simulink model "gm_sampleModel2003_2_sub_sub_sub"  (R2023a)
settings: Solver=VariableStepAuto  StartTime=0.0  StopTime=10.0  RelTol=1e-3
libraries: hdlsllib x7, simulink x2
settings Model: Creator=user1  LastModifiedBy=user1
settings OptimizationCC: BlockReduction=off  ConditionallyExecuteInputs=off
settings DebuggingCC: InheritedTsInSrcMsg=none

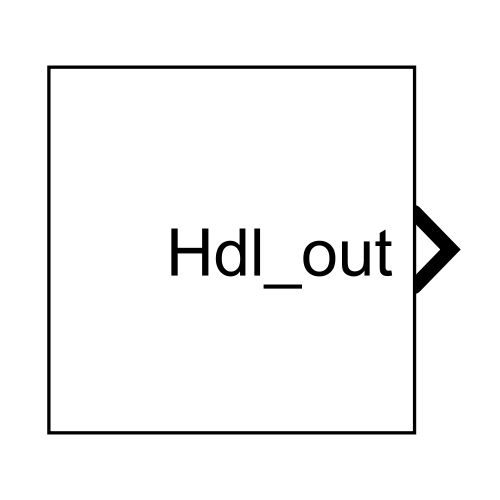
[thumbnail: Simulink's stored preview of the top-level diagram]
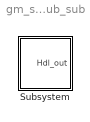
== system gm_sampleModel2003_2_sub_sub_sub ==
  Subsystem : Subsystem

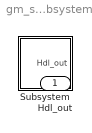
== system gm_sampleModel2003_2_sub_sub_sub/Subsystem ==
  Subsystem : Subsystem
  Hdl_out : Outport  OutDataTypeStr=uint8

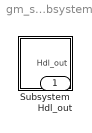
== system gm_sampleModel2003_2_sub_sub_sub/Subsystem/Subsystem ==
  Subsystem : Subsystem
  Hdl_out : Outport  OutDataTypeStr=uint8

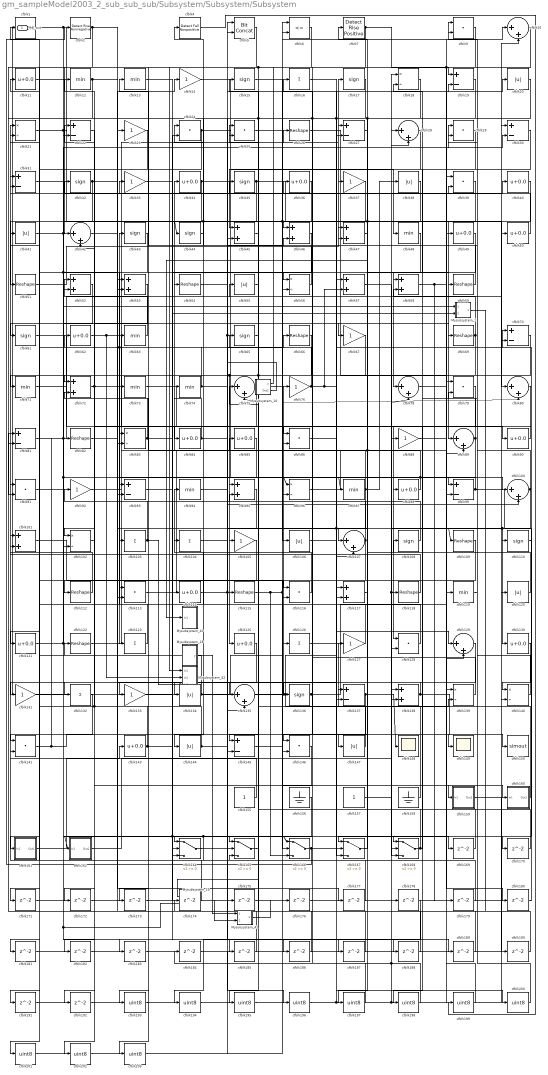
== system gm_sampleModel2003_2_sub_sub_sub/Subsystem/Subsystem/Subsystem ==
  Mysubsystem_1 : Subsystem  TreatAsAtomicUnit=on  RTWFcnName=Mysubsystem_1
      settings: RTWFcnNameOpts=User specified  RTWFileNameOpts=Use function name
  Mysubsystem_10 : Subsystem  TreatAsAtomicUnit=on  RTWFcnName=Mysubsystem_10
      settings: RTWFcnNameOpts=User specified  RTWFileNameOpts=Use function name
  Mysubsystem_28 : Subsystem  TreatAsAtomicUnit=on  RTWFcnName=Mysubsystem_28
      settings: RTWFcnNameOpts=User specified  RTWFileNameOpts=Use function name
  Mysubsystem_29 : Subsystem  TreatAsAtomicUnit=on  RTWFcnName=Mysubsystem_29
      settings: RTWFcnNameOpts=User specified  RTWFileNameOpts=Use function name
  Mysubsystem_40 : Subsystem  TreatAsAtomicUnit=on  RTWFcnName=Mysubsystem_40
      settings: RTWFcnNameOpts=User specified  RTWFileNameOpts=Use function name
  Mysubsystem_41 : Subsystem  TreatAsAtomicUnit=on  RTWFcnName=Mysubsystem_41
      settings: RTWFcnNameOpts=User specified  RTWFileNameOpts=Use function name
  Mysubsystem_42 : Subsystem  TreatAsAtomicUnit=on  RTWFcnName=Mysubsystem_42
      settings: RTWFcnNameOpts=User specified  RTWFileNameOpts=Use function name
  cfblk1 : hdlsllib/Logic and Bit Operations/Compare To Constant  relop=<=  const=3.0  OutDataTypeStr=uint8
  cfblk{10,28,42,75,78,80,89,100,107,129,135} (11 alike) : Sum  Inputs=|++  OutDataTypeStr=uint8
  cfblk{45..47,52..53,57..58,72,95,101,117,138} (12 alike) : Sum  OutDataTypeStr=uint8
  cfblk{18,21,56,83,96,102,139..140} (8 alike) : Product  Inputs=*/  OutDataTypeStr=uint8  RndMeth=Zero  SaturateOnIntegerOverflow=on
  cfblk{16,103..104,123,126,132} (6 alike) : Sum  Inputs=+  OutDataTypeStr=uint8
  cfblk{14,23,33,37,67,76,88,92,105,127,131,133} (12 alike) : Gain  OutDataTypeStr=uint8
  cfblk{20,38,41,55,106,120,134,144,147} (9 alike) : Abs  OutDataTypeStr=uint8  SaturateOnIntegerOverflow=off
  cfblk{15,17,32,35,43..44,61,65,108,110,136} (11 alike) : Signum
  cfblk{26,51,54,59,66,69,82,109,112,115,118,122} (12 alike) : Reshape
  cfblk{11,34,36,40,49..50,62,84..85,90,98,114,121,125,130,143} (16 alike) : Bias  Bias=0.0  SaturateOnIntegerOverflow=off
  cfblk{9,24..25,29,39,79,86,91,113,116,128,141,146} (13 alike) : DotProduct  OutDataTypeStr=uint8
  cfblk{12..13,48,63,71,73..74,94,97,119} (10 alike) : MinMax  OutDataTypeStr=uint8
  cfblk{19,22,27,30..31,70,81,93,99,137,145} (11 alike) : Sum  Inputs=+-  OutDataTypeStr=uint8
  cfblk148 : Scope
  cfblk149 : Scope
  cfblk150 : ToWorkspace  VariableName=simout  SaveFormat=Timeseries  SampleTime=-1
  cfblk155 : Constant  OutDataTypeStr=uint8  SampleTime=-1
  cfblk156 : Ground
  cfblk157 : Constant  OutDataTypeStr=uint8  SampleTime=-1
  cfblk158 : Ground
  cfblk159 : Subsystem
      settings: LibrarySourceBlock=|
      | hdlsllib/Ports &
      | Subsystems/Subsystem
  cfblk160 : Subsystem
      settings: LibrarySourceBlock=|
      | hdlsllib/Ports &
      | Subsystems/Subsystem
  cfblk161 : Subsystem
      settings: LibrarySourceBlock=|
      | hdlsllib/Ports &
      | Subsystems/Subsystem
  cfblk162 : Subsystem
      settings: LibrarySourceBlock=|
      | hdlsllib/Ports &
      | Subsystems/Subsystem
  cfblk{164..168} (5 alike) : Switch  OutDataTypeStr=uint8  SaturateOnIntegerOverflow=off  InputSameDT=off
  cfblk{169..192} (24 alike) : Delay  SampleTime=1
  cfblk{193..203} (11 alike) : DataTypeConversion  OutDataTypeStr=uint8  SaturateOnIntegerOverflow=off  RndMeth=Floor
  cfblk2 : hdlsllib/Logic and Bit Operations/Detect Rise Nonnegative  vinit=0  OutDataTypeStr=uint8
  cfblk4 : hdlsllib/Logic and Bit Operations/Detect Fall Nonpositive  vinit=0  OutDataTypeStr=uint8
  cfblk5 : hdlsllib/Logic and Bit Operations/Bit Concat  numInputs=2
  cfblk6 : RelationalOperator  Operator=<=  OutDataTypeStr=boolean  InputSameDT=off
  cfblk7 : hdlsllib/Logic and Bit Operations/Detect Rise Positive  vinit=0  OutDataTypeStr=uint8
  Hdl_out : Outport  OutDataTypeStr=uint8
  wires:
  Mysubsystem_41/1(Out1) -> cfblk178/1
  Mysubsystem_29/1(Out1) -> Mysubsystem_41/2(In2)
  Mysubsystem_28/1(y) -> Mysubsystem_41/1(In1)
  Mysubsystem_10/2(Out2) -> cfblk100/1, cfblk20/1
  Mysubsystem_10/1(y) -> Mysubsystem_42/1(In1), cfblk145/1
  Mysubsystem_1/1(Out1) -> cfblk174/1
  cfblk203/1 -> cfblk5/2
  cfblk202/1 -> cfblk5/1
  cfblk146/1 -> cfblk202/1
  cfblk201/1 -> cfblk176/1
  cfblk5/1 -> cfblk201/1
  cfblk200/1 -> cfblk79/2
  cfblk196/1 -> cfblk200/1
  cfblk199/1 -> cfblk79/1
  cfblk4/1 -> cfblk199/1
  cfblk198/1 -> cfblk86/2, cfblk18/1
  cfblk197/1 -> cfblk184/1
  cfblk49/1 -> cfblk197/1
  cfblk184/1 -> cfblk196/1
  cfblk195/1 -> cfblk6/2
  cfblk165/1 -> cfblk195/1
  cfblk194/1 -> cfblk6/1
  cfblk178/1 -> cfblk194/1
  cfblk193/1 -> cfblk118/1, cfblk78/2, cfblk120/1, cfblk57/1
  cfblk192/1 -> cfblk165/2
  cfblk191/1 -> cfblk139/1
  cfblk109/1 -> cfblk191/1
  cfblk190/1 -> cfblk116/2
  cfblk159/1(Out1) -> cfblk190/1
  cfblk189/1 -> cfblk168/2
  cfblk131/1 -> cfblk189/1
  cfblk188/1 -> cfblk167/2
  cfblk187/1 -> cfblk81/1
  cfblk27/1 -> cfblk187/1
  cfblk186/1 -> cfblk165/3
  cfblk185/1 -> cfblk53/1
  cfblk91/1 -> cfblk185/1
  cfblk183/1 -> cfblk140/2
  cfblk182/1 -> cfblk30/1
  cfblk105/1 -> cfblk182/1
  cfblk181/1 -> cfblk117/1
  cfblk23/1 -> cfblk181/1
  cfblk180/1 -> cfblk70/2
  cfblk179/1 -> cfblk141/2
  cfblk177/1 -> cfblk75/1
  cfblk176/1 -> cfblk96/2
  cfblk175/1 -> cfblk39/1
  cfblk164/1 -> cfblk175/1
  cfblk174/1 -> cfblk1/1
  cfblk173/1 -> cfblk89/2
  cfblk129/1 -> cfblk173/1
  cfblk172/1 -> cfblk24/2
  cfblk171/1 -> cfblk10/2
  cfblk132/1 -> cfblk171/1
  cfblk170/1 -> cfblk95/2
  cfblk110/1 -> cfblk170/1
  cfblk169/1 -> cfblk18/2
  cfblk57/1 -> cfblk169/1
  cfblk101/1 -> cfblk166/2
  cfblk65/1 -> cfblk15/1
  cfblk58/1 -> cfblk179/1, cfblk180/1
  cfblk6/1 -> cfblk193/1
  cfblk29/1 -> cfblk58/1
  cfblk36/1 -> cfblk52/2
  cfblk74/1 -> cfblk62/1, cfblk135/2
  cfblk160/1(Out1) -> cfblk32/1
  cfblk158/1 -> cfblk137/1
  cfblk41/1 -> cfblk69/1, cfblk30/2
  cfblk83/1 -> cfblk166/1, cfblk186/1, cfblk72/2
  cfblk54/1 -> cfblk110/1
  cfblk138/1 -> cfblk150/1, cfblk136/1
  cfblk55/1 -> cfblk25/1
  cfblk67/1 -> cfblk72/1
  cfblk104/1 -> cfblk46/2
  cfblk22/1 -> cfblk102/1
  cfblk127/1 -> cfblk104/1
  cfblk14/1 -> cfblk48/1
  cfblk108/1 -> cfblk35/1
  cfblk15/1 -> cfblk90/1
  cfblk119/1 -> cfblk29/1
  cfblk28/1 -> cfblk45/1
  cfblk144/1 -> cfblk122/1, cfblk31/1, cfblk27/1
  cfblk73/1 -> cfblk129/2
  cfblk145/1 -> cfblk9/2
  cfblk114/1 -> cfblk29/2, cfblk188/1
  cfblk12/1 -> cfblk23/1, cfblk22/2
  cfblk10/1 -> cfblk75/2, cfblk91/2
  cfblk93/1 -> cfblk164/2
  cfblk13/1 -> cfblk67/1
  cfblk115/1 -> cfblk159/1(In1), cfblk80/2, cfblk166/3
  cfblk123/1 -> cfblk41/1
  cfblk45/1 -> cfblk165/1
  cfblk125/1 -> cfblk141/1
  cfblk9/1 -> cfblk61/1, cfblk99/2
  cfblk116/1 -> cfblk94/1
  cfblk47/1 -> cfblk147/1
  cfblk71/1 -> cfblk50/1
  cfblk168/1 -> cfblk65/1, cfblk108/1
  cfblk82/1 -> cfblk14/1
  cfblk69/1 -> Mysubsystem_29/1(In1), cfblk103/1, cfblk58/2
  cfblk84/1 -> cfblk66/1, cfblk74/1
  cfblk75/1 -> cfblk99/1, cfblk192/1
  cfblk20/1 -> cfblk146/1
  cfblk78/1 -> cfblk10/1
  cfblk21/1 -> cfblk183/1, Mysubsystem_29/2(In2), cfblk46/1
  cfblk167/1 -> cfblk37/1
  cfblk31/1 -> cfblk114/1
  cfblk147/1 -> cfblk127/1
  cfblk16/1 -> cfblk168/1, cfblk109/1
  cfblk37/1 -> cfblk51/1
  cfblk92/1 -> cfblk85/1
  cfblk76/1 -> cfblk19/2, cfblk57/2, cfblk63/1, cfblk31/2
  cfblk32/1 -> cfblk102/2, cfblk177/1
  cfblk140/1 -> cfblk9/1
  cfblk33/1 -> cfblk59/1
  cfblk118/1 -> cfblk101/2
  cfblk94/1 -> cfblk100/2
  cfblk141/1 -> cfblk149/1, cfblk82/1
  cfblk130/1 -> cfblk140/1
  cfblk139/1 -> cfblk16/1
  cfblk95/1 -> cfblk133/1
  cfblk89/1 -> cfblk33/1, cfblk167/3
  cfblk143/1 -> Mysubsystem_1/2(In2), cfblk42/2
  cfblk62/1 -> Mysubsystem_42/2(In2), cfblk115/1
  cfblk157/1 -> cfblk28/2
  cfblk11/1 -> cfblk97/1, cfblk164/3, cfblk53/2
  cfblk61/1 -> cfblk86/1
  cfblk90/1 -> cfblk83/1
  cfblk162/1(Out1) -> cfblk138/2
  cfblk81/1 -> cfblk55/1, cfblk36/1
  cfblk70/1 -> cfblk71/1
  cfblk155/1 -> cfblk101/1
  cfblk79/1 -> cfblk198/1
  cfblk7/1 -> cfblk56/1, cfblk19/1
  cfblk102/1 -> cfblk132/1
  cfblk39/1 -> cfblk44/1, cfblk56/2
  cfblk133/1 -> cfblk39/2
  cfblk98/1 -> cfblk73/1, cfblk47/1, cfblk96/1
  cfblk24/1 -> cfblk117/2, cfblk83/2
  cfblk72/1 -> cfblk54/1, cfblk22/1
  cfblk34/1 -> cfblk138/1, cfblk203/1
  cfblk100/1 -> cfblk130/1, cfblk128/2, cfblk47/2
  cfblk137/1 -> cfblk148/1, cfblk146/2
  cfblk136/1 -> cfblk88/1, Hdl_out/1
  cfblk96/1 -> cfblk28/1
  cfblk117/1 -> cfblk7/1
  cfblk113/1 -> cfblk40/1
  cfblk86/1 -> cfblk98/1
  cfblk50/1 -> cfblk11/1
  cfblk43/1 -> cfblk131/1
  cfblk63/1 -> cfblk52/1
  cfblk40/1 -> Mysubsystem_40/1(In1), cfblk161/1(In1)
  cfblk134/1 -> cfblk21/2, cfblk126/1
  cfblk48/1 -> cfblk78/1
  cfblk88/1 -> cfblk160/1(In1)
  cfblk80/1 -> cfblk128/1
  cfblk52/1 -> cfblk121/1
  cfblk166/1 -> cfblk2/1, cfblk70/1
  cfblk99/1 -> cfblk167/1, cfblk93/1
  cfblk53/1 -> cfblk112/1
  cfblk59/1 -> cfblk4/1
  cfblk56/1 -> cfblk13/1
  cfblk106/1 -> cfblk129/1
  cfblk46/1 -> cfblk123/1
  cfblk103/1 -> Mysubsystem_42/3(In3), cfblk12/1
  cfblk25/1 -> cfblk106/1
  cfblk18/1 -> cfblk116/1, cfblk145/2, cfblk27/2
  cfblk30/1 -> cfblk105/1
  cfblk42/1 -> cfblk164/1
  cfblk112/1 -> cfblk91/1
  cfblk66/1 -> cfblk95/1, cfblk93/2
  cfblk107/1 -> cfblk25/2, cfblk172/1
  cfblk120/1 -> cfblk92/1
  cfblk26/1 -> cfblk119/1
  cfblk85/1 -> cfblk125/1
  cfblk156/1 -> cfblk21/1, cfblk162/1(In1)
  cfblk135/1 -> cfblk139/2, cfblk107/2, cfblk76/1
  cfblk51/1 -> cfblk17/1
  cfblk38/1 -> cfblk134/1
  cfblk44/1 -> cfblk24/1
  cfblk161/1(Out1) -> cfblk143/1
  cfblk128/1 -> cfblk43/1
  cfblk19/1 -> cfblk107/1, cfblk81/2
  cfblk126/1 -> cfblk49/1
  cfblk35/1 -> cfblk144/1, cfblk113/1, cfblk80/1
  cfblk17/1 -> cfblk84/1, cfblk135/1
  cfblk1/1 -> cfblk89/1, cfblk45/2
  cfblk122/1 -> cfblk26/1
  cfblk121/1 -> Mysubsystem_1/1(In1), cfblk168/3
  cfblk97/1 -> cfblk34/1, cfblk38/1, cfblk113/2
  cfblk2/1 -> cfblk42/1, cfblk137/2

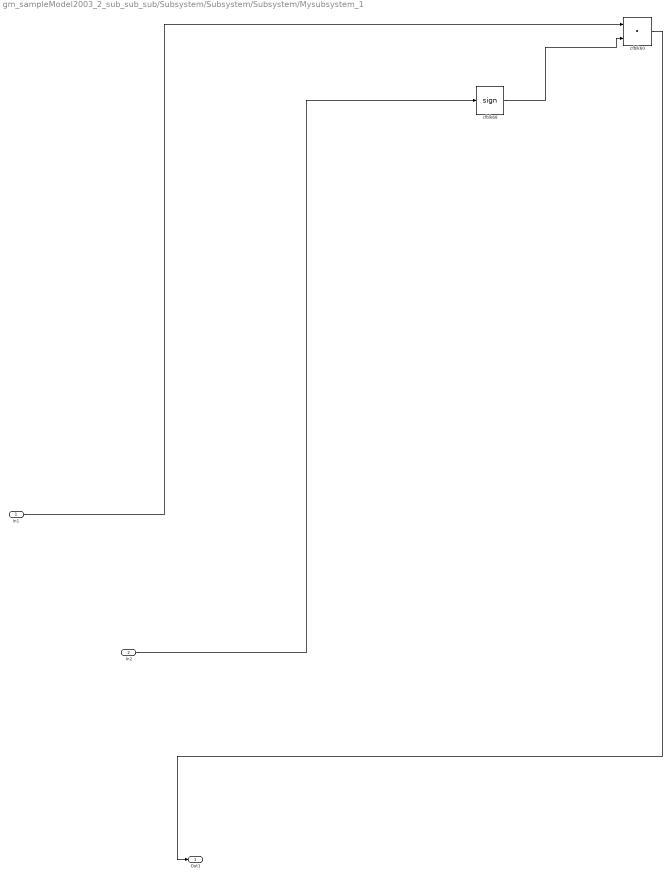
== system gm_sampleModel2003_2_sub_sub_sub/Subsystem/Subsystem/Subsystem/Mysubsystem_1 ==
  In1 : Inport
  In2 : Inport  Port=2
  cfblk60 : DotProduct  OutDataTypeStr=Inherit: Inherit via internal rule
  cfblk68 : Signum
  Out1 : Outport
  wires:
  cfblk68/1 -> cfblk60/2
  In1/1 -> cfblk60/1
  cfblk60/1 -> Out1/1
  In2/1 -> cfblk68/1

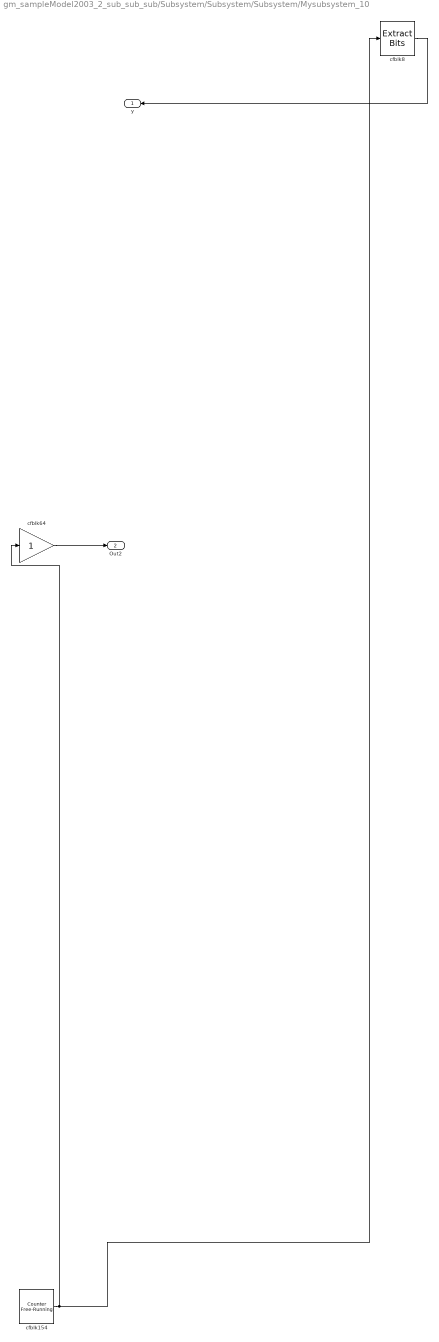
== system gm_sampleModel2003_2_sub_sub_sub/Subsystem/Subsystem/Subsystem/Mysubsystem_10 ==
  cfblk154 : hdlsllib/Sources/Counter Free-Running  NumBits=16  tsamp=-1
  cfblk64 : Gain
  cfblk8 : simulink/Logic and Bit Operations/Extract Bits  bitsToExtract=Upper half  numBits=8  bitIdxRange=[0 7]  outScalingMode=Preserve fixed-point scaling
      settings: LibrarySourceBlock=|
      | hdlsllib/Logic and Bit
      | Operations/Extract Bits
  y : Outport
  Out2 : Outport  Port=2
  wires:
  cfblk64/1 -> Out2/1
  cfblk8/1 -> y/1
  cfblk154/1 -> cfblk8/1, cfblk64/1

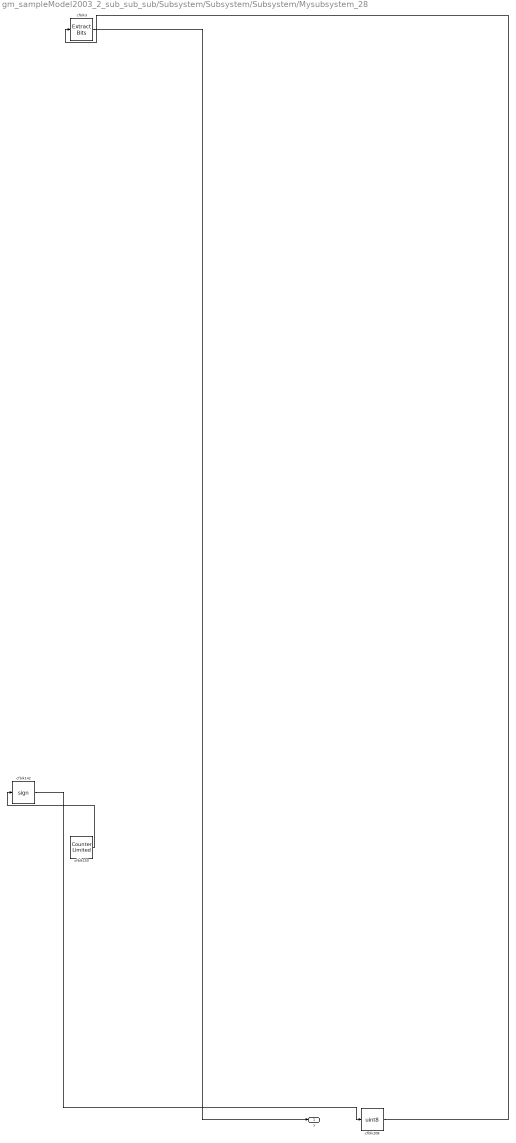
== system gm_sampleModel2003_2_sub_sub_sub/Subsystem/Subsystem/Subsystem/Mysubsystem_28 ==
  cfblk142 : Signum
  cfblk153 : hdlsllib/Sources/Counter Limited  uplimit=7  tsamp=-1
  cfblk208 : DataTypeConversion  OutDataTypeStr=uint8  SaturateOnIntegerOverflow=off  RndMeth=Floor
  cfblk3 : simulink/Logic and Bit Operations/Extract Bits  bitsToExtract=Upper half  numBits=8  bitIdxRange=[0 7]  outScalingMode=Preserve fixed-point scaling
      settings: LibrarySourceBlock=|
      | hdlsllib/Logic and Bit
      | Operations/Extract Bits
  y : Outport
  wires:
  cfblk142/1 -> cfblk208/1
  cfblk208/1 -> cfblk3/1
  cfblk3/1 -> y/1
  cfblk153/1 -> cfblk142/1

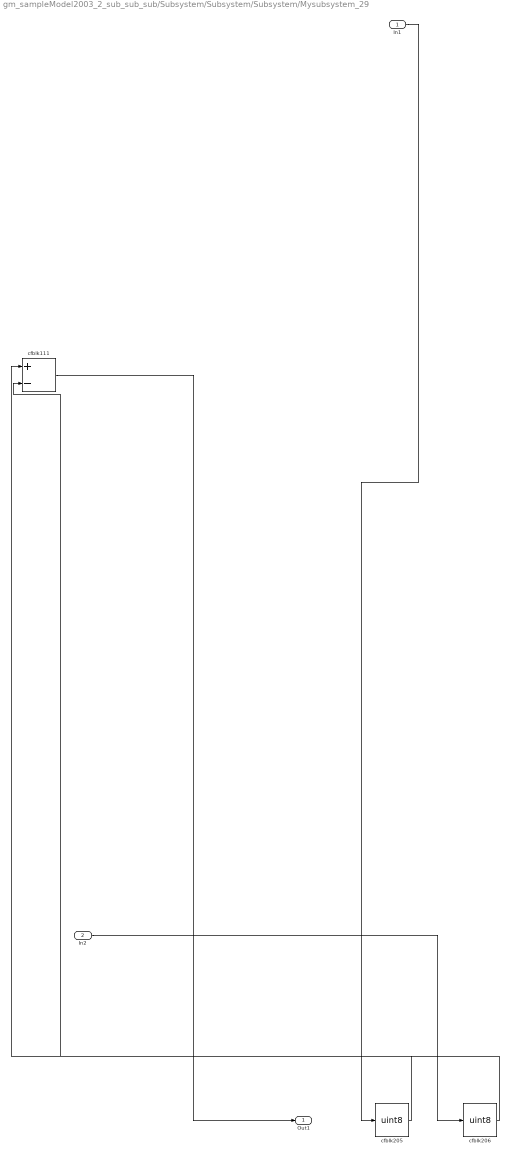
== system gm_sampleModel2003_2_sub_sub_sub/Subsystem/Subsystem/Subsystem/Mysubsystem_29 ==
  In1 : Inport
  In2 : Inport  Port=2
  cfblk111 : Sum  Inputs=+-
  cfblk205 : DataTypeConversion  OutDataTypeStr=uint8  SaturateOnIntegerOverflow=off  RndMeth=Floor
  cfblk206 : DataTypeConversion  OutDataTypeStr=uint8  SaturateOnIntegerOverflow=off  RndMeth=Floor
  Out1 : Outport
  wires:
  cfblk206/1 -> cfblk111/2
  In2/1 -> cfblk206/1
  In1/1 -> cfblk205/1
  cfblk205/1 -> cfblk111/1
  cfblk111/1 -> Out1/1

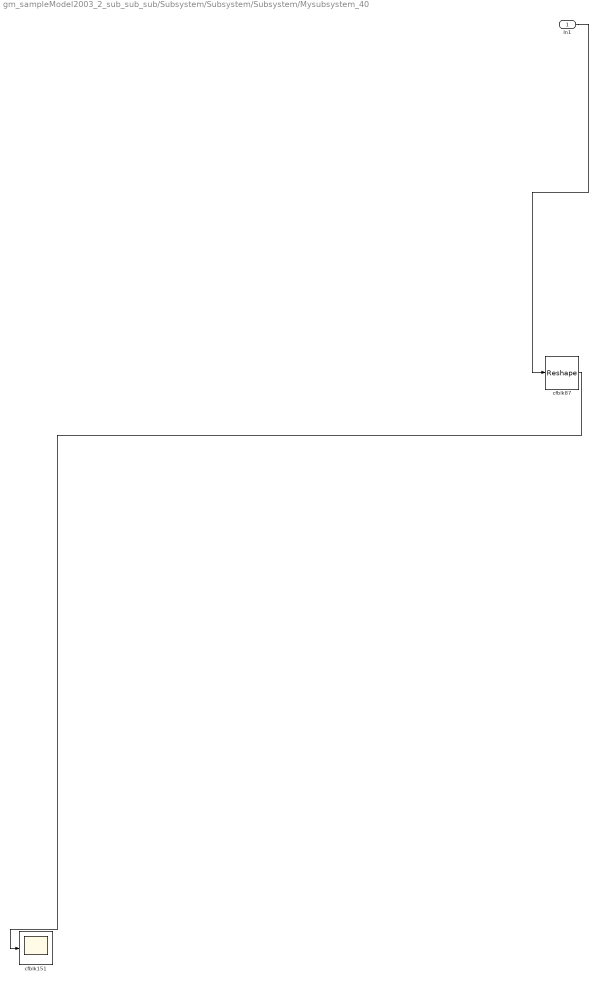
== system gm_sampleModel2003_2_sub_sub_sub/Subsystem/Subsystem/Subsystem/Mysubsystem_40 ==
  In1 : Inport
  cfblk151 : Scope
  cfblk87 : Reshape
  wires:
  In1/1 -> cfblk87/1
  cfblk87/1 -> cfblk151/1

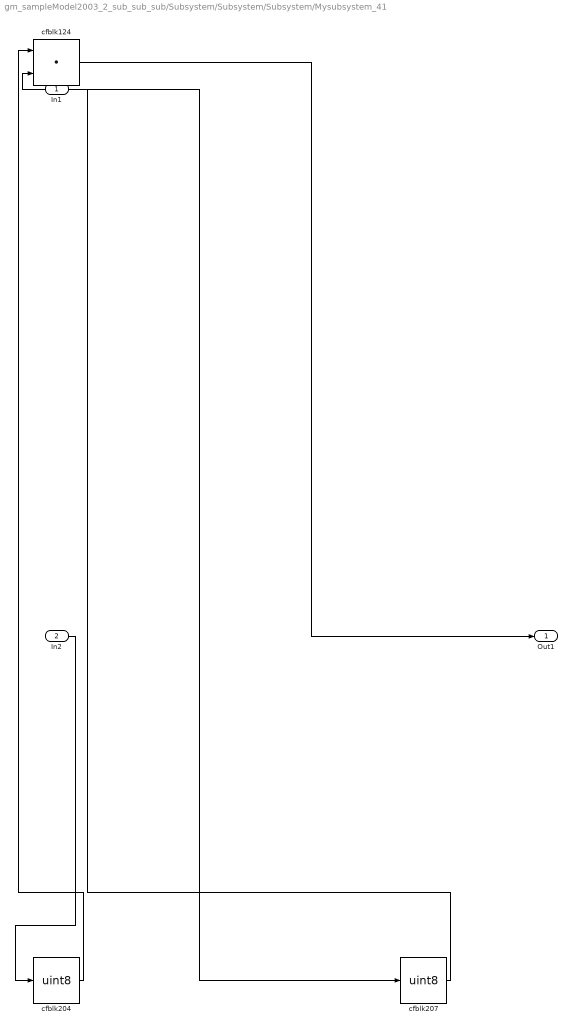
== system gm_sampleModel2003_2_sub_sub_sub/Subsystem/Subsystem/Subsystem/Mysubsystem_41 ==
  In1 : Inport
  In2 : Inport  Port=2
  cfblk124 : DotProduct  OutDataTypeStr=Inherit: Inherit via internal rule
  cfblk204 : DataTypeConversion  OutDataTypeStr=uint8  SaturateOnIntegerOverflow=off  RndMeth=Floor
  cfblk207 : DataTypeConversion  OutDataTypeStr=uint8  SaturateOnIntegerOverflow=off  RndMeth=Floor
  Out1 : Outport
  wires:
  In1/1 -> cfblk207/1
  cfblk207/1 -> cfblk124/2
  In2/1 -> cfblk204/1
  cfblk204/1 -> cfblk124/1
  cfblk124/1 -> Out1/1

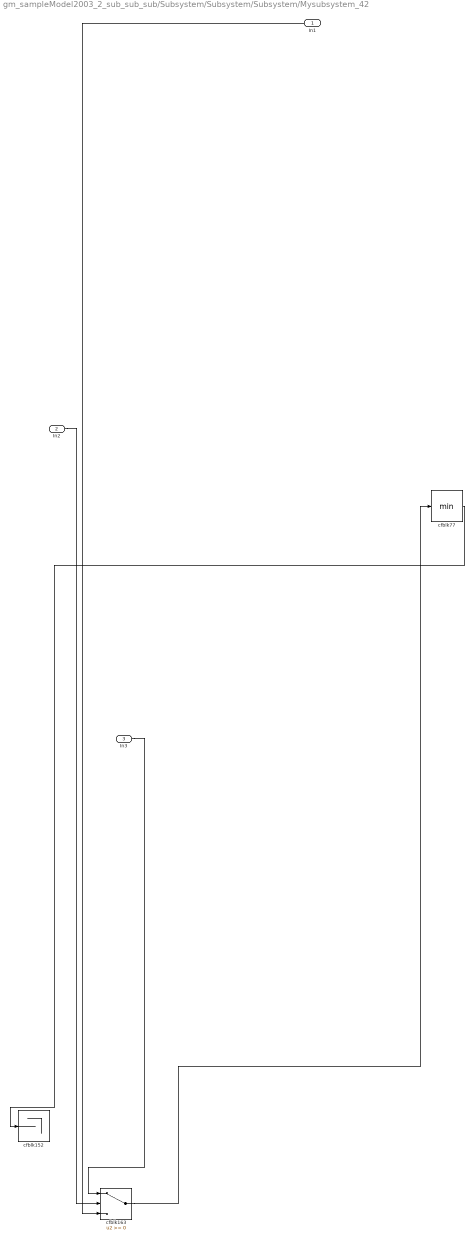
== system gm_sampleModel2003_2_sub_sub_sub/Subsystem/Subsystem/Subsystem/Mysubsystem_42 ==
  In1 : Inport
  In2 : Inport  Port=2
  In3 : Inport  Port=3
  cfblk152 : Terminator
  cfblk163 : Switch  SaturateOnIntegerOverflow=off  InputSameDT=off
  cfblk77 : MinMax
  wires:
  cfblk163/1 -> cfblk77/1
  In3/1 -> cfblk163/1
  cfblk77/1 -> cfblk152/1
  In1/1 -> cfblk163/3
  In2/1 -> cfblk163/2

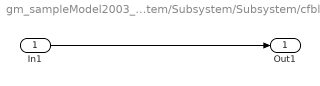
== system gm_sampleModel2003_2_sub_sub_sub/Subsystem/Subsystem/Subsystem/cfblk159 ==
  In1 : Inport
  Out1 : Outport
  wires:
  In1/1 -> Out1/1

== system gm_sampleModel2003_2_sub_sub_sub/Subsystem/Subsystem/Subsystem/cfblk160 ==
  In1 : Inport
  Out1 : Outport
  wires:
  In1/1 -> Out1/1

== system gm_sampleModel2003_2_sub_sub_sub/Subsystem/Subsystem/Subsystem/cfblk161 ==
  In1 : Inport
  Out1 : Outport
  wires:
  In1/1 -> Out1/1

== system gm_sampleModel2003_2_sub_sub_sub/Subsystem/Subsystem/Subsystem/cfblk162 ==
  In1 : Inport
  Out1 : Outport
  wires:
  In1/1 -> Out1/1
